simulink model "simulink_model"  (R2024b)
settings: Solver=ode15s  StartTime=0.0  StopTime=1  MaxStep=1e-2  MinStep=1e-6
values from neighbouring files (symbols this model uses):
  K = [Kred(:,1:5), zeros(4,1), Kred(:,6:end), zeros(4,1)]    [acadosSim.m]    (also in claudeSim.m = zeros(nu, nx); claudeSim_CORRECTED.m = zeros(nu, nx); claudeSim_EXACT_REPLICATION.m; ellipke_casadi.m = K_poly1 - K_poly2 .* log(m1))
  x0 = xLp + [0.001 -0.003 0.04 pi/5 0 0 zeros(1, 6)].'    [acadosSim.m]    (also in claudeSim.m = xEq + [0.001, -0.003, 0.04, pi/5, 0, 0, zeros(1, 6)]'; claudeSim_CORRECTED.m = xEq + [0, 0, 0.002, 0.01, 0, 0, zeros(1, 6)]'; claudeSim_EXACT_REPLICATION.m = xLp + [0.001, -0.003, 0.04, pi/5, 0, 0, zeros(1, 6)]'; compareModels.m = xLp + [0 0.00025 0.0045 0 deg2rad(2) 0 zeros(1, 6)].')
  xLp = [0,0,zEq(1),zeros(1,9)]'    [acadosSim.m]    (also in claudeSim_EXACT_REPLICATION.m = [0, 0, zEq(1), zeros(1,9)]'; compareModels.m; compareModels2.m = [0,0,zEq(1)+0.001,zeros(1,9)]')
settings Model: Creator=halva  LastModifiedBy=halva
settings SolverCC: MaxOrder=4  ConsecutiveZCsStepRelTol=1000*128*eps  MaxConsecutiveZCs=10000  ZeroCrossAlgorithm=Adaptive

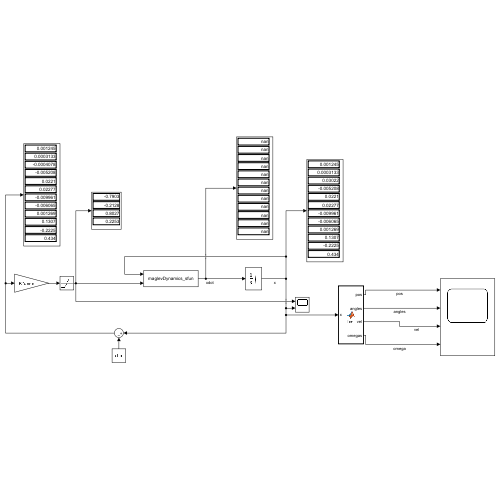
[thumbnail: Simulink's stored preview of the top-level diagram]
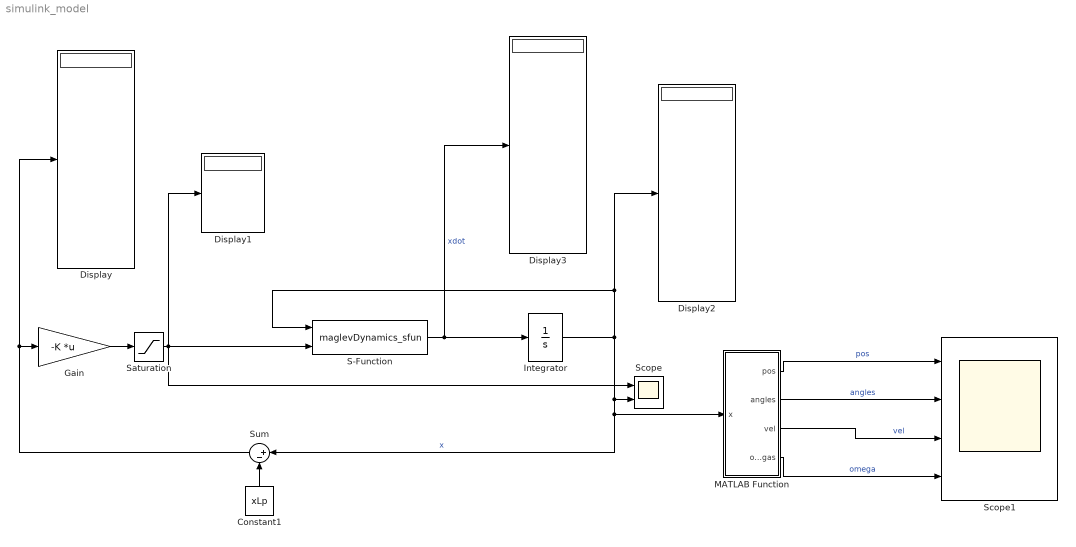
== system simulink_model ==
  Constant1 : Constant  Value=xLp  VectorParams1D=off
  Display{,1..3} (4 alike) : Display
  Gain : Gain  Gain=-K  Multiplication=Matrix(K*u) (u vector)
  Integrator : Integrator  InitialCondition=x0  LimitOutput=on  UpperSaturationLimit=ones(12,1)  LowerSaturationLimit=-ones(12,1)
  MATLAB Function : MATLAB Function  TreatAsAtomicUnit=on
  S-Function : S-Function  FunctionName=maglevDynamics_sfun  SFunctionDeploymentMode=off  EnableBusSupport=off
  Saturation : Saturate  UpperLimit=ones(4,1)*5  LowerLimit=-ones(4,1)*5
  Scope : Scope  NumInputPorts=2
  Scope1 : Scope  NumInputPorts=4
  Sum : Sum  Inputs=|+-
  wires:
  S-Function/1 -> Display3/1, Integrator/1  "xdot"
  Integrator/1 -> Display2/1, S-Function/1, Sum/1, MATLAB Function/1(x), Scope/2  "x"
  Gain/1 -> Saturation/1
  Sum/1 -> Display/1, Gain/1
  Constant1/1 -> Sum/2
  Saturation/1 -> Display1/1, Scope/1, S-Function/2
  MATLAB Function/1(pos) -> Scope1/1  "pos"
  MATLAB Function/2(angles) -> Scope1/2  "angles"
  MATLAB Function/3(vel) -> Scope1/3  "vel"
  MATLAB Function/4(omegas) -> Scope1/4  "omega"

== matlab function simulink_model/MATLAB Function ==
  data: x input; pos output; angles output; vel output; omegas output
function [pos,angles,vel,omegas] = fcn(x)
pos = x(1:3,:);
angles = x(4:5,:);
vel = x(6:9,:);
omegas = x(10:11,:);
